simulink model "SG__MDL_IO104_IO135_DirectCoupling"  (R2022b)
settings: Solver=FixedStepAuto  StartTime=0.0  StopTime=Inf  RelTol=1e-3  EnableMultiTasking=on
model workspace (MAT data in the model file):
  a = 0.28
  ff = 1200
  fi = 150
  tmax = 40
undefined symbols (not defined in the file): Ended, Single
libraries: dspfdesign x6, simulink x4, speedgoatlib_IO135 x3, speedgoatlib_IO104 x3, hdlsllib x2, slrealtimeloglib x1, dspsrcs4 x1
settings Model: SimulationMode=external  Creator=padlewsk  LastModifiedBy=padlewsk
settings SolverCC: ConcurrentTasks=on  AlgebraicLoopSolver=TrustRegion  PositivePriorityOrder=on  AutoInsertRateTranBlk=on
settings DataIOCC: SaveFormat=StructureWithTime
settings OptimizationCC: BlockReduction=off  OptimizeBlockIOStorage=off
settings DebuggingCC: TasksWithSamePriorityMsg=none  UnconnectedInputMsg=warning  UnconnectedOutputMsg=warning  UnconnectedLineMsg=warning
settings HardwareCC: ProdBitPerLong=64  ProdLongLongMode=on  ProdHWDeviceType=Intel->x86-64 (Linux 64)
settings ModelReferenceCC: EnableRefExpFcnMdlSchedulingChecks=on
settings RTWCC: Description=Simulink Real-Time  SystemTargetFile=slrealtime.tlc  TemplateMakefile=slrealtime_default_tmf  Toolchain=Simulink Real-Time Toolchain  BuildConfiguration=Faster Runs  CodeExecutionProfiling=on  TargetLang=C++

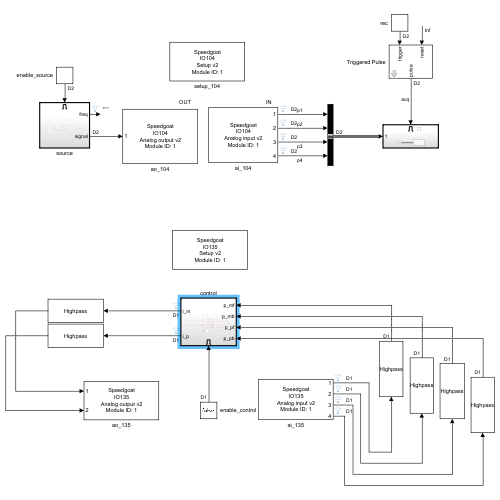
[thumbnail: Simulink's stored preview of the top-level diagram]
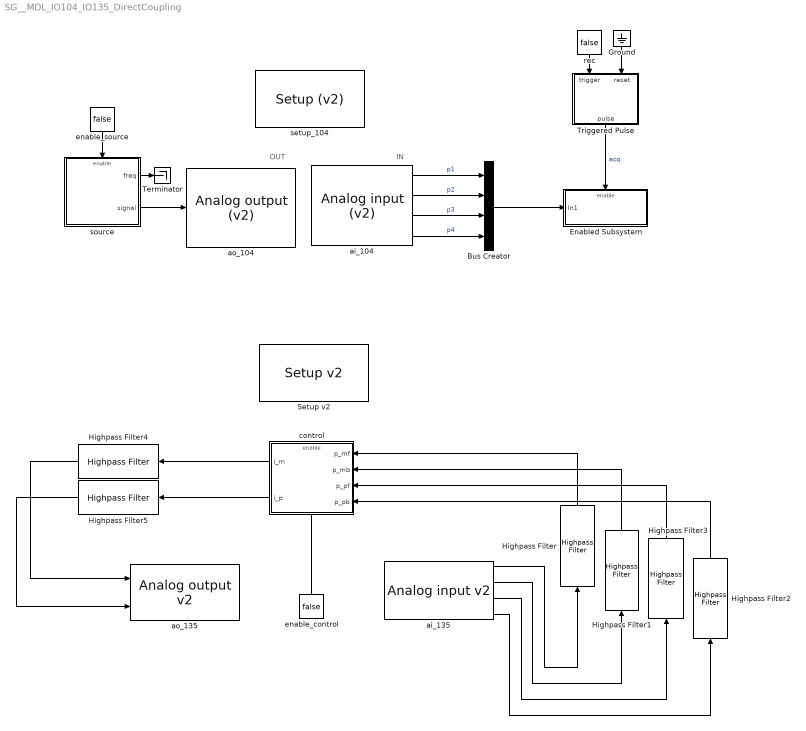
== system SG__MDL_IO104_IO135_DirectCoupling ==
  note: IN
  note: OUT
  Bus Creator : BusCreator  Inputs=4
  Enabled Subsystem : Subsystem  TreatAsAtomicUnit=on
  Ground : Ground
  Highpass Filter{,1..5} (6 alike) : dspfdesign/Highpass Filter  FilterType=IIR  DesignForMinimumOrder=off  FilterOrder=4  StopbandFrequency=1  PassbandFrequency=5  StopbandAttenuation=40  PassbandRipple=0.5  InheritSampleRate=on  SampleRate=44100  SimulateUsing=Interpreted execution  roundingMode=Floor  coeffsDataTypeStr=fixdt(1,16)
  "Setup v2 " : speedgoatlib_IO135/Setup v2   parPciSlot=-1  parModuleId=1  parInterModuleSync=None  parConvClockBaseRate=20MHz  parConvClock1Divider=20000  parConvClock2Divider=20000  parFrameTriggerEnable=off  parFrameTriggerDivider=10  parConvClock1BaseRate=1  parConvClock2BaseRate=1  parFrameTriggerClock=1  parAdcChannels=[1:4]  parAdcRange1=+-5V  parAdcRange2=+-5V  parAdcRange3=+-5V  parAdcRange4=+-5V  parAdcVoltageRange=[1 1 1 1]  parAdcOversampling1=None  parAdcOversampling2=None  parAdcOversampling3=None  parAdcOversampling4=None  parAdcOversamplRate=[1 1 1 1]  parAdcAutoCorrection=on  parAdcContSampling=off  parAdcDmaEnable=off  parAdcDmaClock=Clock 1  parAdcFrameSize_=100  parAdcSampleTime_=-1  parAdcActiveDmaDevices=[1 1 1 1]  parAdcFrameTriggerEnable=0  parAdcFrameSize=100  parAdcSampleTime=0.1  parDacChannels=[1 2]  parDacInitValues=0  parDacReset=1  parDacRange1=+-10V  parDacRange2=+-10V  parDacRange3=+-10V  parDacRange4=+-10V  parDacRange5=+-10V  parDacRange6=+-10V  parDacRange7=+-10V  parDacRange8=+-10V  parDacRange9=+-10V  parDacRange10=+-10V  parDacRange11=+-10V  parDacRange12=+-10V  parDacRange13=+-10V  parDacRange14=+-10V  parDacRange15=+-10V  parDacRange16=+-10V  parDacVoltageRange=[5 5 5 5 5 5 5 5 5 5 5 5 5 5 5 5]  parDacAutoCorrection=on  parDacSyncOut=on  parDacDmaEnable=off  parDacDmaLatency=Until next frame  parDacDmaClock=Clock 1  parDacFrameSize_=100  parDacSampleTime_=-1  parDacActiveDmaDevices=[1 1 1 1]  parDacFrameTriggerEnable=0  parDacFrameSize=100  parDacSampleTime=0.1  parDoChannels=[]  parDoInitValues=0  parDoReset=1  parDiChannels=[]  parDiDebounceEnable=off  parDiDebounceTime=0  parDiDebounceValue=0  parDioPullRefFront=Pull-up 3.3V  parDioPullRefRear=Floating
      settings: SourceProductName=Simulink Real-Time: Speedgoat I/O Blockset
  Terminator : Terminator
  Triggered Pulse : Subsystem  mask(Triggered Pulse){N=4}
      mask prompts: N "Length (N samples)"
      mask help: Generates a single pulse of N samples length
  ai_104 : speedgoatlib_IO104/Analog input (v2)   parModuleId=1  parTs=0.0001  parPciSlot=-1  parAdChannels=[1,2,3,4]  parAdChannelsSorted=[1,2,3,4]  parAdRange1=+-10V  parAdRange2=+-10V  parAdCoupling=Single-Ended  parAdFrameSize=1  parAdUseTrigger=off  parAdClockInitiator=Initiator  parAdSampleTime=9.920634921e-07  parTriggerInitiator=Target  parTriggerRate=4.161015625e-01
      settings: SourceProductName=Simulink Real-Time: Speedgoat I/O Blockset
  ai_135 : speedgoatlib_IO135/Analog input v2   parModuleId=1  parSampleTime=5e-05  parPciSlot=-1  parAdcChannels=[1 2 3 4]  parAdcVoltageRange=[1 1 1 1]  parAdcOversamplRate=[1 1 1 1]  parAdcContSampling=0  parAdcDmaEnable=0  parAdcActiveDmaDevices=[1 1 1 1]  parAdcFrameSize=100
      settings: SourceProductName=Simulink Real-Time: Speedgoat I/O Blockset
  ao_104 : speedgoatlib_IO104/Analog output (v2)   parModuleId=1  parTs=0.0001  parPciSlot=-1  parDaChannels=1  parDaChannelsSorted=1  parDaInitValue=0  parDaReset=1  parDaRange=+-2.5V  parDaFrameSize=1  parDaUseTrigger=off  parDaClockInitiator=Initiator  parDaSampleTime=9.920634921e-07  parTriggerInitiator=Target  parTriggerRate=4.161015625e-01  parAdBlockPresent=1
      settings: SourceProductName=Simulink Real-Time: Speedgoat I/O Blockset
  ao_135 : speedgoatlib_IO135/Analog output v2   parModuleId=1  parSampleTime=5e-05  parPciSlot=-1  parDacChannels=[1 2]  parDacVoltageRange=[5 5 5 5 5 5 5 5 5 5 5 5 5 5 5 5]  parDacInitValues=[0 0]  parDacReset=[1 1]  parDacSyncOut=1  parDacDmaEnable=0  parDacActiveDmaDevices=[1 1 1 1]  parDacDmaLatency=2  parDacFrameSize=100
      settings: SourceProductName=Simulink Real-Time: Speedgoat I/O Blockset
  control : Subsystem
  enable_control : Constant  Value=false  SampleTime=-1
  enable_source : Constant  Value=false  SampleTime=-1
  rec : Constant  Value=false  SampleTime=-1
  setup_104 : speedgoatlib_IO104/Setup (v2)   parPciSlot=-1  parModuleId=1  parTriggerInitiator=Target  parTriggerRate=4.161015625e-01  parCalibrate=off  parAdChannels=[1:4]  parAdRange1=+-10V  parAdRange2=+-10V  parAdCoupling=Single-Ended  parAdUseTrigger=off  parAdFrameSize=1  parAdClockInitiator=Initiator  parAdSampleTime=9.920634921e-07  parDaChannels=[1]  parDaChannelsSorted=1  parDaInitValue=[0]  parDaReset=[1]  parDaRange=+-2.5V  parDaUseTrigger=off  parDaFrameSize=1  parDaClockInitiator=Initiator  parDaSampleTime=9.920634921e-07  parDioByte0Dir=Outputs  parDioByte1Dir=Inputs  parDoChannels=[1:4]  parDoInitValues=[0]  parDoReset=[1]  parDiChannels=[13:16]
      settings: SourceProductName=Simulink Real-Time: Speedgoat I/O Blockset
  source : Subsystem  TreatAsAtomicUnit=on
  wires:
  enable_source/1 -> source/Enable
  ai_104/3 -> Bus Creator/3  "p3"
  ai_104/1 -> Bus Creator/1  "p1"
  ai_104/2 -> Bus Creator/2  "p2"
  enable_control/1 -> control/Enable
  source/2(signal) -> ao_104/1
  ai_104/4 -> Bus Creator/4  "p4"
  Triggered Pulse/1(pulse) -> Enabled Subsystem/Enable  "acq"
  Ground/1 -> Triggered Pulse/2(reset)
  rec/1 -> Triggered Pulse/1(trigger)
  Bus Creator/1 -> Enabled Subsystem/1(In1)
  source/1(freq) -> Terminator/1
  ai_135/1 -> Highpass Filter/1
  ai_135/2 -> Highpass Filter1/1
  ai_135/3 -> Highpass Filter3/1
  ai_135/4 -> Highpass Filter2/1
  control/1(i_m) -> Highpass Filter4/1
  control/2(i_p) -> Highpass Filter5/1
  Highpass Filter/1 -> control/1(p_mf)
  Highpass Filter1/1 -> control/2(p_mb)
  Highpass Filter2/1 -> control/4(p_pb)
  Highpass Filter3/1 -> control/3(p_pf)
  Highpass Filter4/1 -> ao_135/1
  Highpass Filter5/1 -> ao_135/2

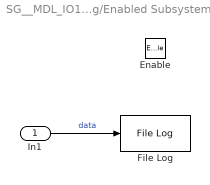
== system SG__MDL_IO104_IO135_DirectCoupling/Enabled Subsystem ==
  In1 : Inport
  Enable : EnablePort
  File Log : slrealtimeloglib/File Log  decimation=1  inputProcessing=Elements as channels (sample based)
  wires:
  In1/1 -> File Log/1  "data"

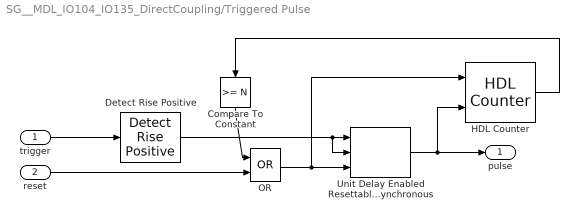
== system SG__MDL_IO104_IO135_DirectCoupling/Triggered Pulse ==
  trigger : Inport
  reset : Inport  Port=2
  Compare To Constant : simulink/Logic and Bit Operations/Compare To Constant  relop=>=  const=N  OutDataTypeStr=boolean
  Detect Rise Positive : simulink/Logic and Bit Operations/Detect Rise Positive  vinit=0  OutDataTypeStr=boolean
  HDL Counter : hdlsllib/Sources/HDL Counter  CountType=Free running  CountInit=1  CountStep=1  CountMax=25  CountFromType=Initial value  CountFrom=1  CountResetPort=on  CountLoadPort=off  CountEnbPort=on  CountDirPort=off  CountHitOutputPort=off  CountDataType=Unsigned  CountWordLen=32  CountFracLen=0  CountSampTime=1
  OR : Logic  Operator=OR  AllPortsSameDT=off  OutDataTypeStr=boolean
  Unit Delay Enabled Resettable Synchronous : hdlsllib/Discrete/Unit Delay Enabled Resettable Synchronous  InitialCondition=0.0  SampleTime=-1
  pulse : Outport  VectorParamsAs1DForOutWhenUnconnected=off
  wires:
  OR/1 -> Unit Delay Enabled Resettable Synchronous/3, HDL Counter/1
  trigger/1 -> Detect Rise Positive/1
  Unit Delay Enabled Resettable Synchronous/1 -> HDL Counter/2, pulse/1
  Compare To Constant/1 -> OR/1
  reset/1 -> OR/2
  Detect Rise Positive/1 -> Unit Delay Enabled Resettable Synchronous/1, Unit Delay Enabled Resettable Synchronous/2
  HDL Counter/1 -> Compare To Constant/1

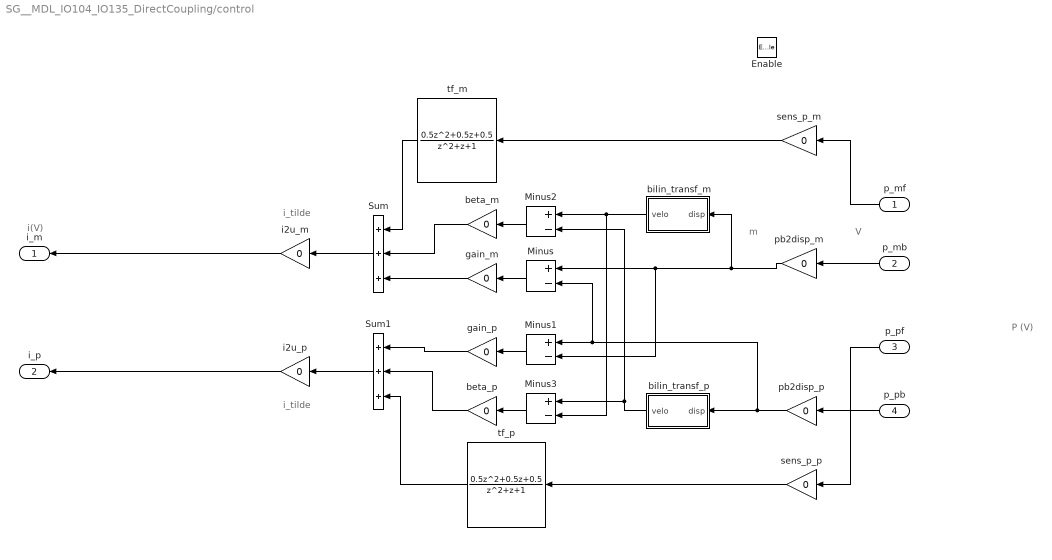
== system SG__MDL_IO104_IO135_DirectCoupling/control ==
  note: m
  note: P (V)
  note: i_tilde
  note: i(V)
  note: i_tilde
  note: V
  p_mf : Inport
  p_mb : Inport  Port=2
  p_pf : Inport  Port=3
  p_pb : Inport  Port=4
  Enable : EnablePort
  Minus{,1..3} (4 alike) : Sum  Inputs=+-
  Sum : Sum  Inputs=+++
  Sum1 : Sum  Inputs=+++
  beta_m : Gain  Gain=0
  beta_p : Gain  Gain=0
  bilin_transf_m : Subsystem
  bilin_transf_p : Subsystem
  gain_m : Gain  Gain=0
  gain_p : Gain  Gain=0
  i2u_m : Gain  Gain=0
  i2u_p : Gain  Gain=0
  pb2disp_m : Gain  Gain=0
  pb2disp_p : Gain  Gain=0
  sens_p_m : Gain  Gain=0
  sens_p_p : Gain  Gain=0
  tf_m : DiscreteTransferFcn  Numerator="[0.5         0.5         0.5]"  Denominator="[1  1  1]"
  tf_p : DiscreteTransferFcn  Numerator="[0.5         0.5         0.5]"  Denominator="[1  1  1]"
  i_m : Outport
  i_p : Outport  Port=2
  wires:
  p_mb/1 -> pb2disp_m/1
  p_pf/1 -> sens_p_p/1
  p_pb/1 -> pb2disp_p/1
  p_mf/1 -> sens_p_m/1
  Minus/1 -> gain_m/1
  Minus1/1 -> gain_p/1
  sens_p_m/1 -> tf_m/1
  sens_p_p/1 -> tf_p/1
  Sum/1 -> i2u_m/1
  Sum1/1 -> i2u_p/1
  tf_m/1 -> Sum/1
  gain_m/1 -> Sum/3
  tf_p/1 -> Sum1/3
  gain_p/1 -> Sum1/1
  i2u_m/1 -> i_m/1
  i2u_p/1 -> i_p/1
  pb2disp_p/1 -> Minus1/1, Minus/2, bilin_transf_p/1(disp)
  pb2disp_m/1 -> bilin_transf_m/1(disp), Minus/1, Minus1/2
  Minus2/1 -> beta_m/1
  beta_p/1 -> Sum1/2
  Minus3/1 -> beta_p/1
  bilin_transf_p/1(velo) -> Minus2/2, Minus3/1
  bilin_transf_m/1(velo) -> Minus3/2, Minus2/1
  beta_m/1 -> Sum/2

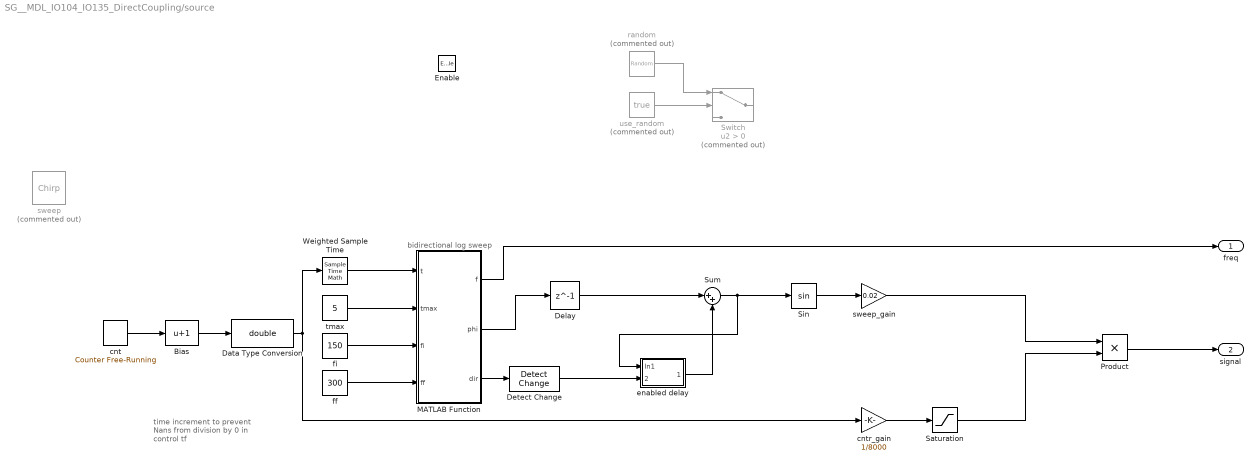
== system SG__MDL_IO104_IO135_DirectCoupling/source ==
  note: bidirectional log sweep
  note: time increment to prevent Nans from division by 0 in control tf
  Enable : EnablePort  StatesWhenEnabling=reset
  Bias : Bias  Bias=1  SaturateOnIntegerOverflow=off
  Data Type Conversion : DataTypeConversion  OutDataTypeStr=double  SaturateOnIntegerOverflow=off  RndMeth=Floor
  Delay : Delay  DelayLength=1
  Detect Change : simulink/Logic and Bit Operations/Detect Change  vinit=false  OutDataTypeStr=boolean
  MATLAB Function : MATLAB Function  TreatAsAtomicUnit=on
  Product : Product
  Saturation : Saturate  UpperLimit=1  LowerLimit=0
  Sin : Trigonometry
  Sum : Sum  Inputs=|++
  Switch : Switch  Commented=on  Criteria=u2 > Threshold  SaturateOnIntegerOverflow=off  InputSameDT=off
  Weighted Sample Time : SampleTimeMath  TsampMathOp=*
  cnt : simulink/Sources/Counter Free-Running  NumBits=32  tsamp=-1
  cntr_gain : Gain  Gain=1/8000  ParamDataTypeStr=double
  enabled delay : Subsystem
  ff : Constant  Value=300
  fi : Constant  Value=150
  random : RandomNumber  Commented=on  Variance=0.5  SampleTime=3.5e-05
  sweep : dspsrcs4/Chirp  Commented=on  sweep=Logarithmic  mode=Bidirectional  f0=150  f1=1200  t1=10  Tsweep=20  phase=0  Ts=3.5e-05  spf=1  datatype=Double  OutputFrames=off
  sweep_gain : Gain  Gain=0.02
  tmax : Constant  Value=5
  use_random : Constant  Commented=on  Value=true  SampleTime=-1
  freq : Outport  OutputWhenDisabled=reset  InitialOutput=0  VectorParamsAs1DForOutWhenUnconnected=off
  signal : Outport  Port=2  OutputWhenDisabled=reset  InitialOutput=0  VectorParamsAs1DForOutWhenUnconnected=off
  wires:
  use_random/1 -> Switch/2
  random/1 -> Switch/1
  sweep_gain/1 -> Product/1
  cntr_gain/1 -> Saturation/1
  Product/1 -> signal/1
  MATLAB Function/2(phi) -> Delay/1
  Saturation/1 -> Product/2
  Weighted Sample Time/1 -> MATLAB Function/1(t)
  Data Type Conversion/1 -> cntr_gain/1, Weighted Sample Time/1
  MATLAB Function/1(f) -> freq/1
  Sin/1 -> sweep_gain/1
  MATLAB Function/3(dir) -> Detect Change/1
  Detect Change/1 -> enabled delay/2(enable)
  Delay/1 -> Sum/1
  enabled delay/1(Out1) -> Sum/2
  Sum/1 -> enabled delay/1(In1), Sin/1
  cnt/1 -> Bias/1
  Bias/1 -> Data Type Conversion/1
  ff/1 -> MATLAB Function/4(ff)
  tmax/1 -> MATLAB Function/2(tmax)
  fi/1 -> MATLAB Function/3(fi)

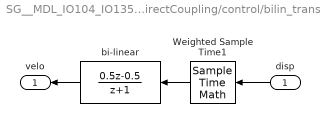
== system SG__MDL_IO104_IO135_DirectCoupling/control/bilin_transf_m ==
  disp : Inport
  Weighted Sample Time1 : SampleTimeMath  TsampMathOp=/
  "bi-linear " : DiscreteTransferFcn  Numerator=[0.5, -0.5]  Denominator=[1, 1]
  velo : Outport
  wires:
  disp/1 -> Weighted Sample Time1/1
  Weighted Sample Time1/1 -> "bi-linear "/1
  "bi-linear "/1 -> velo/1

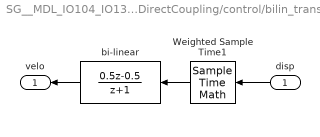
== system SG__MDL_IO104_IO135_DirectCoupling/control/bilin_transf_p ==
  disp : Inport
  Weighted Sample Time1 : SampleTimeMath  TsampMathOp=/
  "bi-linear " : DiscreteTransferFcn  Numerator=[0.5, -0.5]  Denominator=[1, 1]
  velo : Outport
  wires:
  disp/1 -> Weighted Sample Time1/1
  Weighted Sample Time1/1 -> "bi-linear "/1
  "bi-linear "/1 -> velo/1

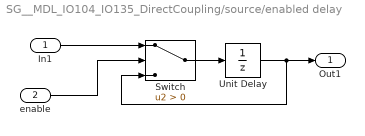
== system SG__MDL_IO104_IO135_DirectCoupling/source/enabled delay ==
  In1 : Inport
  enable : Inport  Port=2
  Switch : Switch  Criteria=u2 > Threshold  SaturateOnIntegerOverflow=off  InputSameDT=off
  Unit Delay : UnitDelay  SampleTime=-1  HasFrameUpgradeWarning=on
  Out1 : Outport
  wires:
  Unit Delay/1 -> Switch/3, Out1/1
  Switch/1 -> Unit Delay/1
  In1/1 -> Switch/1
  enable/1 -> Switch/2

== matlab function SG__MDL_IO104_IO135_DirectCoupling/source/MATLAB Function ==
  data: f output; t input; tmax input; phi output; dir output; fi input; ff input
function [f, phi, dir] = fcn(t, tmax, fi, ff)
%tmax is the time at which the maximum frequency is reached

t = mod(t, 2*tmax);

if t < tmax
    % up
    dir = 1;
    
    
    % linear (CF wikipedia)
%     phi = 2*pi*(0.5*(ff - fi)*t^2/tmax + fi*t);
%     f = fi + (ff - fi)*t/tmax;
    
    % logarithmic %%% https://en.wikipedia.org/wiki/Chirp
    k = log((ff/fi)^(1/tmax));
    phi = 2*pi*fi*(exp(k*t) - 1)/k;
    f = fi*exp(k*t);
else
    % down
    dir = -1;
    
    
    % linear (CF wikipedia)
%     phi = 2*pi*(0.5*(fi - ff)*(t-tmax)^2/tmax + ff*(t-tmax)); % linear
%     f = ff + (fi - ff)*(t - tmax)/tmax;
    
    % logarithmic
    k = log((fi/ff)^(1/tmax));
    phi = 2*pi*ff*(exp(k*(t - tmax)) - 1)/k;
    f = ff*exp(k*(t-tmax));
end

phi = mod(phi, 2*pi);
